simulink model "mod2_ilatest"  (Simulink 8.1)
settings: Solver=FixedStepDiscrete  StartTime=0.0  StopTime=swpctrl.trantime  RelTol=1e-3
undefined symbols (not defined in the file): DACctrl, Fs, modctrl, sinamp, sinfreq
libraries: simulink x3, dspsigops x3, dspsrcs4 x2
settings Model: Creator=amyles  LastModifiedBy=amyles
settings DataIOCC: LimitDataPoints=off  MaxDataPoints=50000
settings DebuggingCC: StrictBusMsg=Warning
settings SFSimCC: SimParseCustomCode=off

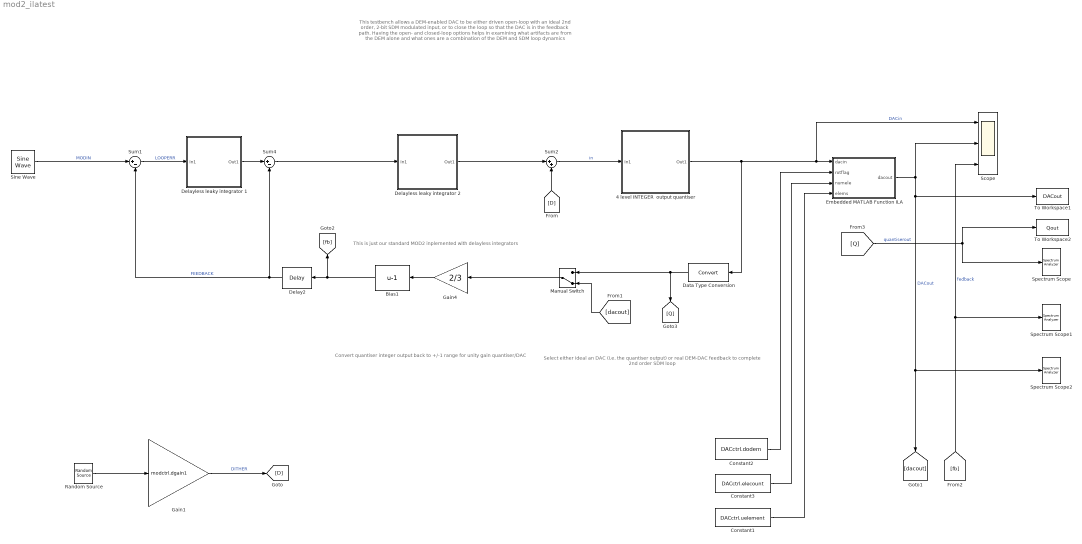
== system mod2_ilatest ==
  note: Convert quantiser integer output
      | back  to +/-1 range for
      | unity gain quantiser/DAC
  note: Select either ideal an DAC
      | (i.e. the quantiser output) or real
      | DEM-DAC feedback to complete
      | 2nd order SDM loop
  note: This testbench allows a DEM-enabled DAC to be either driven open-loop with an ideal 2nd order, 2-bit SDM modulated input,
      | or to close the loop so that the DAC is in the feedback path. Having the open- and closed-loop options helps in
      | examining what artifacts are from the DEM alone and what ones are a combination of the DEM and SDM loop dynamics
  note: This is just our standard MOD2 inplemented with delayless integrators
  4 level INTEGER  output quantiser : Subsystem
  Bias1 : Bias  Bias=-1
  Constant1 : Constant  Value=DACctrl.uelement  SampleTime=1/Fs
  Constant2 : Constant  Value=DACctrl.dodem  SampleTime=1/Fs
  Constant3 : Constant  Value=DACctrl.elecount  SampleTime=1/Fs
  Data Type Conversion : DataTypeConversion
  Delay2 : dspsigops/Delay  InputProcessing=Inherited (this choice will be removed - see release notes)  dly_unit=Samples  delay=1  ic_detail=off  dif_ic_for_ch=off  dif_ic_for_dly=off  ic=0  reset_popup=None
  Delayless leaky integrator 1 : Subsystem
  Delayless leaky integrator 2 : Subsystem
  Embedded MATLAB Function ILA : MATLAB Function  TreatAsAtomicUnit=on
  Gain1 : Gain  Gain=modctrl.dgain1
      settings: AttributesFormatString=Dither level adjust
  Gain4 : Gain  Gain=2/3
      settings: AttributesFormatString=Integrator leakage
  Manual Switch : ManualSwitch  CurrentSetting=0
  Random Source : dspsrcs4/Random Source  SrcType=Uniform  NormMethod=Ziggurat  CltLength=12  MinVal=-1  MaxVal=1  MeanVal=0  VarVal=1  RepMode=Not repeatable  rawSeed=1  IsInherit=off  SampMode=Discrete  SampTime=1/Fs  SampFrame=1  DataType=Double  OutComplex=Real
      settings: AttributesFormatString=Dither source
  Scope : Scope  NumInputPorts=3
      settings: YMin=-5~-5~-5  YMax=5~5~5
  Sine Wave : dspsrcs4/Sine Wave  Amplitude=sinamp  Frequency=sinfreq  Phase=0  SampleMode=Discrete  OutComplex=Real  CompMethod=Trigonometric fcn  TableSize=Speed  SampleTime=1/Fs  SamplesPerFrame=1  ResetState=Restart at time zero  dataType=double  wordLen=16  udDataType=sfix(16)  fracBitsMode=Best precision  numFracBits=15  OutDataTypeStr=double  LastOutDataTypeStr=double
  Spectrum Scope : SpectrumAnalyzer
      settings: CopyFcn=scopeextensions.ScopeBlock.callback(gcbh, 'onBlockCopy', gcbh);  DeleteFcn=scopeextensions.ScopeBlock.callback(gcbh, 'onBlockDelete');  PreSaveFcn=scopeextensions.ScopeBlock.callback(gcbh, 'onModelSave');  NameChangeFcn=scopeextensions.ScopeBlock.callback(gcbh, 'onBlockRename');  CloseFcn=scopeextensions.ScopeBlock.callback(gcbh, 'onBlockClose');  PreDeleteFcn=scopeextensions.ScopeBlock.callback(gcbh, 'onBlockPreDelete');
  Spectrum Scope1 : SpectrumAnalyzer
      settings: CopyFcn=scopeextensions.ScopeBlock.callback(gcbh, 'onBlockCopy', gcbh);  DeleteFcn=scopeextensions.ScopeBlock.callback(gcbh, 'onBlockDelete');  PreSaveFcn=scopeextensions.ScopeBlock.callback(gcbh, 'onModelSave');  NameChangeFcn=scopeextensions.ScopeBlock.callback(gcbh, 'onBlockRename');  CloseFcn=scopeextensions.ScopeBlock.callback(gcbh, 'onBlockClose');  PreDeleteFcn=scopeextensions.ScopeBlock.callback(gcbh, 'onBlockPreDelete');
  Spectrum Scope2 : SpectrumAnalyzer
      settings: CopyFcn=scopeextensions.ScopeBlock.callback(gcbh, 'onBlockCopy', gcbh);  DeleteFcn=scopeextensions.ScopeBlock.callback(gcbh, 'onBlockDelete');  PreSaveFcn=scopeextensions.ScopeBlock.callback(gcbh, 'onModelSave');  NameChangeFcn=scopeextensions.ScopeBlock.callback(gcbh, 'onBlockRename');  CloseFcn=scopeextensions.ScopeBlock.callback(gcbh, 'onBlockClose');  PreDeleteFcn=scopeextensions.ScopeBlock.callback(gcbh, 'onBlockPreDelete');
  Sum1 : Sum  Inputs=|+-
      settings: AttributesFormatString=Modulator input\nloop servo error (input - fbk)
  Sum2 : Sum  Inputs=|++
  Sum4 : Sum  Inputs=|+-
  To Workspace1 : ToWorkspace  VariableName=DACout  SampleTime=-1
  To Workspace2 : ToWorkspace  VariableName=Qout  SampleTime=-1
  wires:
  Sum1/1 -> Delayless leaky integrator 1/1(In1)  "LOOPERR"
  Delay2/1 -> Sum1/2, Sum4/2  "FEEDBACK"
  Sine Wave/1 -> Sum1/1  "MODIN"
  Sum4/1 -> Delayless leaky integrator 2/1(In1)
  Random Source/1 -> Gain1/1
  Embedded MATLAB Function ILA/1(dacout) -> Scope/2, To Workspace1/1, [dacout], Spectrum Scope2/1  "DACout"
  4 level INTEGER  output quantiser/1(Out1) -> Scope/1, Embedded MATLAB Function ILA/1(dacin), Data Type Conversion/1  "DACin"
  Constant2/1 -> Embedded MATLAB Function ILA/2(rotflag)
  Constant3/1 -> Embedded MATLAB Function ILA/3(numele)
  Constant1/1 -> Embedded MATLAB Function ILA/4(elems)
  Data Type Conversion/1 -> Manual Switch/1, [Q]
  Gain1/1 -> [D]  "DITHER"
  [D] -> Sum2/2
  Manual Switch/1 -> Gain4/1
  [dacout] -> Manual Switch/2
  Bias1/1 -> Delay2/1, [fb]
  Gain4/1 -> Bias1/1
  [Q] -> To Workspace2/1, Spectrum Scope/1  "quantiserout"
  Sum2/1 -> 4 level INTEGER  output quantiser/1(In1)  "in"
  Delayless leaky integrator 1/1(Out1) -> Sum4/1
  Delayless leaky integrator 2/1(Out1) -> Sum2/1
  [fb] -> Scope/3, Spectrum Scope1/1  "fedback"

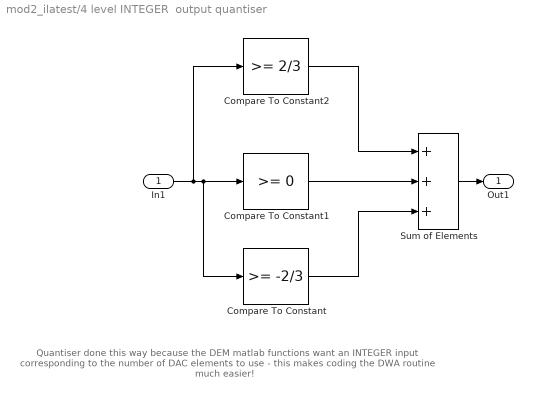
== system mod2_ilatest/4 level INTEGER  output quantiser ==
  note: Quantiser done this way because the DEM matlab
      | functions want an INTEGER input corresponding to
      | the number of DAC elements to use - this makes coding the
      | DWA routine much easier!
  In1 : Inport
  Compare To Constant : simulink/Logic and Bit Operations/Compare To Constant  relop=>=  const=-2/3  OutDataTypeStr=uint8
  Compare To Constant1 : simulink/Logic and Bit Operations/Compare To Constant  relop=>=  const=0  OutDataTypeStr=uint8
  Compare To Constant2 : simulink/Logic and Bit Operations/Compare To Constant  relop=>=  const=2/3  OutDataTypeStr=uint8
  Sum of Elements : Sum  Inputs=+++
  Out1 : Outport
  wires:
  Compare To Constant1/1 -> Sum of Elements/2
  Compare To Constant2/1 -> Sum of Elements/1
  Compare To Constant/1 -> Sum of Elements/3
  In1/1 -> Compare To Constant/1, Compare To Constant1/1, Compare To Constant2/1
  Sum of Elements/1 -> Out1/1

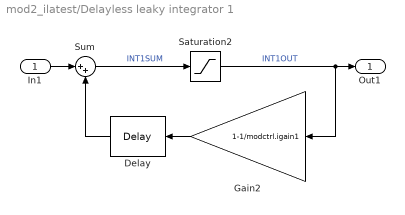
== system mod2_ilatest/Delayless leaky integrator 1 ==
  In1 : Inport
  Delay : dspsigops/Delay  InputProcessing=Inherited (this choice will be removed - see release notes)  dly_unit=Samples  delay=1  ic_detail=off  dif_ic_for_ch=off  dif_ic_for_dly=off  ic=0  reset_popup=None
  Gain2 : Gain  Gain=1-1/modctrl.igain1
      settings: AttributesFormatString=Integrator leakage
  Saturation2 : Saturate  UpperLimit=modctrl.isat1  LowerLimit=-(modctrl.isat1)
  Sum : Sum  Inputs=|++
      settings: AttributesFormatString=Integrator summer
  Out1 : Outport
  wires:
  Delay/1 -> Sum/2
  Sum/1 -> Saturation2/1  "INT1SUM"
  Gain2/1 -> Delay/1
  Saturation2/1 -> Gain2/1, Out1/1  "INT1OUT"
  In1/1 -> Sum/1

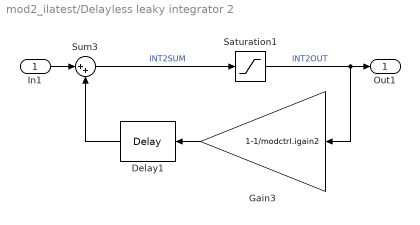
== system mod2_ilatest/Delayless leaky integrator 2 ==
  In1 : Inport
  Delay1 : dspsigops/Delay  InputProcessing=Inherited (this choice will be removed - see release notes)  dly_unit=Samples  delay=1  ic_detail=off  dif_ic_for_ch=off  dif_ic_for_dly=off  ic=0  reset_popup=None
  Gain3 : Gain  Gain=1-1/modctrl.igain2
      settings: AttributesFormatString=Integrator leakage
  Saturation1 : Saturate  UpperLimit=modctrl.isat2  LowerLimit=-(modctrl.isat2)
  Sum3 : Sum  Inputs=|++
      settings: AttributesFormatString=Integrator summer
  Out1 : Outport
  wires:
  Delay1/1 -> Sum3/2
  Sum3/1 -> Saturation1/1  "INT2SUM"
  Gain3/1 -> Delay1/1
  Saturation1/1 -> Gain3/1, Out1/1  "INT2OUT"
  In1/1 -> Sum3/1

== matlab function Embedded MATLAB Function ILA ==
  data: dacin input double; dacout output double; rotflag input double; numele input double; elems input double
function dacout = DAC(dacin, rotflag, numele, elems)
%#eml

% ------------------ Begin Copyright notice -----------------------------
%
% COPYRIGHT AND PROPERTY OF DIALOG SEMICONDUCTOR, 2012.
%
% THIS COPYRIGHT NOTICE MUST NOT BE REMOVED OR MODIFIED.
%
% Commerical use is not permitted.
%
% Installation on systems available for use in any way by commercial users
% is not permitted.
%
% Permission for use is granted by Dialog Semiconductor only for the
% purposes of teaching or studying course ELEE11080/PGEE11110 "Sigma
% Delta Data Converters" (or any renamed variant or descendant of
% this course) at the University of Edinburgh.
%
% Personal copying and/or modification is permitted only by students and
% teaching staff of course PGEE11110 solely for the purposes of delivering
% or studying course PGEE11110.
%
% All permissions for use of this or modified copies are revoked upon
% ceasation of teaching duties or completion or de-enrollment for any
% reason from course PGEE11110.
%
% ------------------- End Copyright notice ------------------------------

% This function assumes a MATLAB workspace structures exists called
% DACctrl with contents:
%
% DACctrl.dodem = DEM enable flag, 0 = no ILA, 1 = apply ILA
% DACctrl.elecount = number fo unit elements in the DAC
% DACctrl.uelement(1) = size of first unit element
% ...
% DACctrl.uelement(elecount) = size of last unit element


persistent ila_pointer; % Need a persistent rotator state

dacplus1 = dacin+1; % Quantiser starts at 0, MATLAB array indices at 1...

% static memory cannot be dynamic, so just allocate enough for
% any realistic DAC. Edit this function if you *really* need more
% than 100 DAC elements...

if isempty(ila_pointer)
    ila_pointer = ones(1,100);    % initialise per-code indices
end

if (rotflag == 0)
    ila_pointer(1,dacplus1) = 1;    % reset if not rotating
end

dacout = 0.0;
ipt = ila_pointer(1,dacplus1);
for indx = 1:1:dacin
    dacout = dacout + elems(ipt);
    ipt = mod(ipt, numele) + 1;
% Above line is a faster way of saying...
%     ila_pointer(dacplus1) = ila_pointer(dacplus1) + 1;
%     if (ila_pointer(dacplus1) > numele)
%         ila_pointer(dacplus1) = 1;
%    end
end
ila_pointer(1,dacplus1) = ipt;

end
